simulink model "V_2_0_SystemsmModelling_ModifyAirCon"  (R2020a)
settings: Solver=ode23t  StartTime=0.0  StopTime=20000  MaxStep=2000.0  RelTol=1e-3
undefined symbols (not defined in the file or in its folder): building_height, building_length, building_width, Discrete, duct_area, fan_flow_rate_table, fan_setting_table, floor_conductivity, floor_heat_transfer_coeff_internal, floor_thickness, ground_temperature, initial_temperature, roof_conductivity, roof_density, roof_heat_transfer_coeff_external, roof_heat_transfer_coeff_internal, roof_specific_heat, roof_thickness, sigbuilder_block, Time, wall_conductivity, wall_density, wall_heat_transfer_coeff_external, wall_heat_transfer_coeff_internal, wall_specific_heat, wall_thickness
libraries: fl_lib x93, nesl_utility x16, simulink x1, ctrlSharedLib x1
(part 1 of 3)
settings Model: Creator=denni  LastModifiedBy=denni

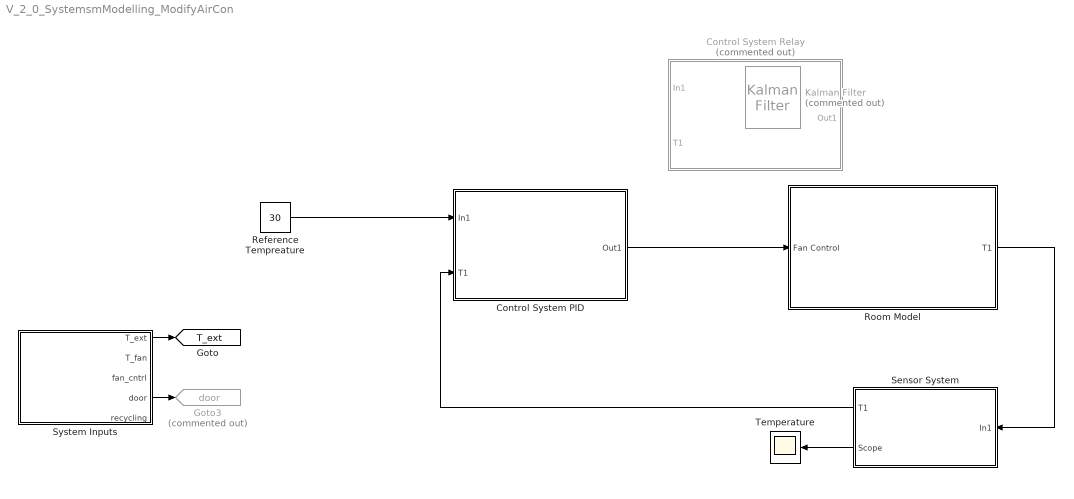
== system V_2_0_SystemsmModelling_ModifyAirCon ==
  Control System PID : Subsystem
  Control System Relay : Subsystem  Commented=on
  Goto3 : Goto  Commented=on  GotoTag=door  TagVisibility=global
  Kalman Filter : ctrlSharedLib/Kalman Filter  Commented=on  TimeDomain=Discrete-Time  UseCurrentEstimator=on  ModelSource=LTI State-Space Variable  ModelSourceVariable=ss(0.95,1,1,0,1)  A=0.95  B=1  C=1  D=0  NumberOfStates=1  NumberOfInputs=1  NumberOfOutputs=1  InitialEstimateSource=Dialog  X0=0  P0=10  UseK=off  UseGH=off  NumberOfProcessNoiseInputs=1  G=1  TimeInvariantG=on  H=0  TimeInvariantH=on  Q=0.05  TimeInvariantQ=on  R=1  TimeInvariantR=on  N=0  TimeInvariantN=on  AddInputPort=on  AddEnablePort=off  OutputEstimatedY=off  OutputP=off  Ts=-1
  "Reference Tempreature " : Constant  Value=30
  "Room Model " : Subsystem
  Sensor System : Subsystem
  System Inputs : Subsystem  Tag=STV Subsys  LoadFcn=sigbuilder_block('load');  StartFcn=sigbuilder_block('start');  StopFcn=sigbuilder_block('stop');  ClipboardFcn=sigbuilder_block('clipboard');  mask(Sigbuilder block){tuvar=[0:10]}
      mask help: Simulink:masks:SigbuilderBlock_MD
      mask init:
      | if ~strcmp(get_param(bdroot(gcbh),'SimulationStatus'),'stopped') tuvar = sigbuilder_block('maskInit'); end
      settings: CopyFcn=sigbuilder_block('copy');  DeleteFcn=sigbuilder_block('delete');  ModelCloseFcn=sigbuilder_block('modelClose');  PreSaveFcn=sigbuilder_block('preSave');  PauseFcn=sigbuilder_block('pause');  ContinueFcn=sigbuilder_block('continue');  NameChangeFcn=sigbuilder_block('namechange');  OpenFcn=sigbuilder_block('open',[334.8 172.8 550.8 361.2 ]);  CloseFcn=sigbuilder_block('close');
      mask Display: plot(0, 0, 100, 100,[2, 2, 32, 32, 2], [68, 8, 8, 68, 68],[32, 2], [38, 38], [32, 19, 2],[53, 60, 44], [32, 17, 17, 2],[16, 16, 31, 31]);txt = getActiveGroup(gcbh);text(2, 100, txt,'verticalAlignment', 'top');
  Temperature : Scope
  tag scope: T_ext=global
  wires:
  System Inputs/4(door) -> Goto3/1
  System Inputs/1(T_ext) -> [T_ext]
  "Room Model "/1(T1) -> Sensor System/1(In1)
  Sensor System/1(T1) -> Control System PID/2(T1)
  Sensor System/2(Scope) -> Temperature/1
  "Reference Tempreature "/1 -> Control System PID/1(In1)
  Control System PID/1(Out1) -> "Room Model "/1(Fan Control)

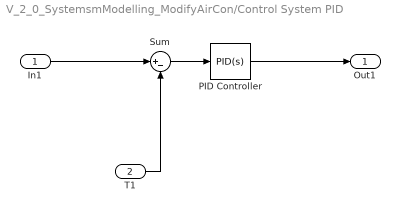
== system V_2_0_SystemsmModelling_ModifyAirCon/Control System PID ==
  In1 : Inport
  T1 : Inport  Port=2
  PID Controller : simulink/Continuous/PID Controller  Controller=PID  Form=Parallel  TimeDomain=Continuous-time  UseExternalTs=off  SampleTime=-1  IntegratorMethod=Forward Euler  FilterMethod=Forward Euler  ControllerParametersSource=internal  P=-0.718298192525533  I=-0.00178286353180639  D=22.2787509507692  UseFilter=on  N=0.00872543218655351  TunerSelectOption=Transfer Function Based (PID Tuner App)  InitialConditionSource=internal  InitialConditionForIntegrator=0  InitialConditionForFilter=0  DifferentiatorICPrevScaledInput=0  ExternalReset=none  TrackingMode=off  Kt=1  LimitOutput=off  UpperSaturationLimit=inf  LowerSaturationLimit=-inf  LinearizeAsGain=on  AntiWindupMode=none  Kb=1  POutMin=[]  POutMax=[]  IOutMin=[]  IOutMax=[]  DOutMin=[]  DOutMax=[]  NOutMin=[]  NOutMax=[]  SumOutMin=[]  SumOutMax=[]  SaturationOutMin=[]  SaturationOutMax=[]  PParamMin=[]  PParamMax=[]  IParamMin=[]  IParamMax=[]  DParamMin=[]  DParamMax=[]  NParamMin=[]  NParamMax=[]  KbParamMin=[]  KbParamMax=[]  KtParamMin=[]  KtParamMax=[]  KbOutMin=[]  KbOutMax=[]  KtOutMin=[]  KtOutMax=[]  IntegratorOutMin=[]  IntegratorOutMax=[]  FilterOutMin=[]  FilterOutMax=[]  SumI1OutMin=[]  SumI1OutMax=[]  SumI2OutMin=[]  SumI2OutMax=[]  SumI3OutMin=[]  SumI3OutMax=[]  SumI4OutMin=[]  SumI4OutMax=[]  SumDOutMin=[]  SumDOutMax=[]  DifferentiatorOutMin=[]  DifferentiatorOutMax=[]  FilterDiffOutCoefMin=[]  FilterDiffOutCoefMax=[]  ReciprocalOutMin=[]  ReciprocalOutMax=[]  SumDenOutMin=[]  SumDenOutMax=[]  SumNumOutMin=[]  SumNumOutMax=[]  DivideOutMin=[]  DivideOutMax=[]  UdiffTsProdOutMin=[]  UdiffTsProdOutMax=[]  NTsProdOutMin=[]  NTsProdOutMax=[]  UintegralTsProdOutMin=[]  UintegralTsProdOutMax=[]  UngainTsProdOutMin=[]  UngainTsProdOutMax=[]  IntegratorContinuousStateAttributes=''  IntegratorStateMustResolveToSignalObject=off  IntegratorRTWStateStorageClass=Auto  FilterContinuousStateAttributes=''  FilterStateMustResolveToSignalObject=off  FilterRTWStateStorageClass=Auto  ParallelPVariant=InternalParameters  IdealPVariant=Disabled  IVariant=InternalParameters  DVariant=InternalParameters  IntegratorVariant=Continuous  SatVariant=Disabled  AWVariant=Passthrough  PCopyVariant=Disabled  TRVariant=Disabled  FdbkBlocksVariant=Forward  IdealPFdbkVariant=Disabled  SatFdbkVariant=Disabled  DerivativeFilterVariant=ContFilter  NVariant=InternalParameters  NCopyVariant=Disabled  FilterICVariant=InternalICsFilter  IntegratorICVariant=InternalICs  ExternalResetVariant=Disabled  TRSumVariant=Passthrough  SumFdbkVariant=Disabled  SumVariant=Sum_PID  TsampFilterVariant=InternalTs  TsampNgainVariant=Passthrough  TsampIntegralVariant=Passthrough
  Sum : Sum  Inputs=|+-
  Out1 : Outport
  wires:
  In1/1 -> Sum/1
  T1/1 -> Sum/2
  Sum/1 -> PID Controller/1
  PID Controller/1 -> Out1/1

== system V_2_0_SystemsmModelling_ModifyAirCon/Control System Relay ==
  In1 : Inport
  T1 : Inport  Port=2
  Relay : Relay  OnSwitchValue=2  OffSwitchValue=-2
  Sum : Sum  Inputs=|-+
  Out1 : Outport
  wires:
  Sum/1 -> Relay/1
  Relay/1 -> Out1/1
  T1/1 -> Sum/2
  In1/1 -> Sum/1

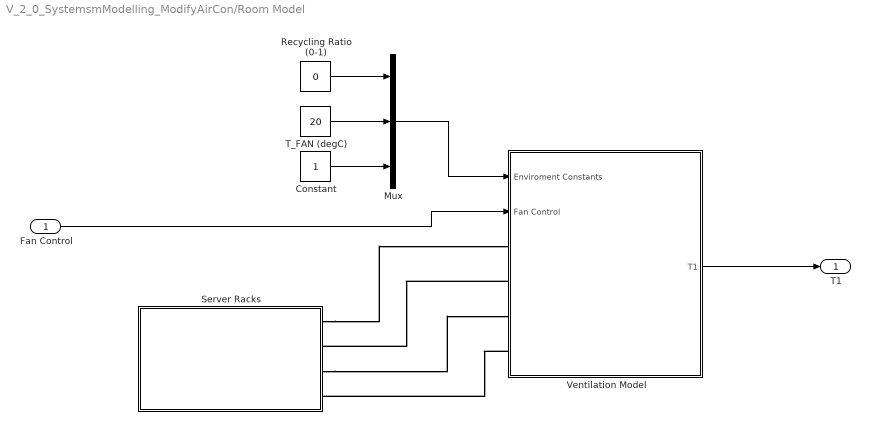
== system V_2_0_SystemsmModelling_ModifyAirCon/Room Model  ==
  Fan Control : Inport
  Constant : Constant
  Mux : Mux  Inputs=3
  Recycling Ratio (0-1) : Constant  Value=0
  Server Racks : Subsystem
  T_FAN (degC) : Constant  Value=20
  Ventilation Model : Subsystem
  T1 : Outport
  wires:
  Constant/1 -> Mux/3
  Recycling Ratio (0-1)/1 -> Mux/1
  T_FAN (degC)/1 -> Mux/2
  Mux/1 -> Ventilation Model/1(Enviroment Constants)
  Fan Control/1 -> Ventilation Model/2(Fan Control)
  Ventilation Model/1(T1) -> T1/1
  connections:
  Server Racks/LConn1 -- Ventilation Model/LConn1
  Ventilation Model/LConn2 -- Server Racks/LConn2
  Server Racks/LConn3 -- Ventilation Model/LConn3
  Ventilation Model/LConn4 -- Server Racks/LConn4

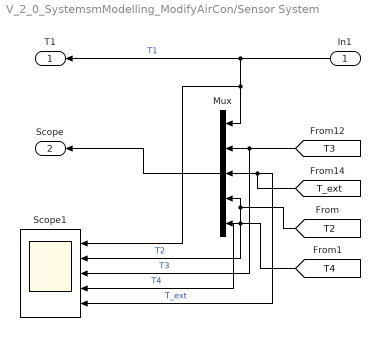
== system V_2_0_SystemsmModelling_ModifyAirCon/Sensor System ==
  In1 : Inport
  Mux : Mux  Inputs=5
  Scope1 : Scope  NumInputPorts=5
  T1 : Outport
  Scope : Outport  Port=2
  wires:
  [T3] -> Scope1/3, Mux/2  "T3"
  Mux/1 -> Scope/1
  [T_ext] -> Mux/3, Scope1/5  "T_ext"
  In1/1 -> Mux/1, Scope1/1, T1/1  "T1"
  [T4] -> Scope1/4, Mux/5  "T4"
  [T2] -> Mux/4, Scope1/2  "T2"

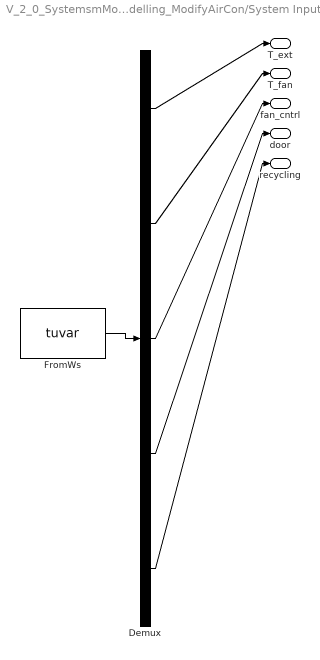
== system V_2_0_SystemsmModelling_ModifyAirCon/System Inputs ==
  Demux : Demux  Tag=STV Demux  Outputs=5
      settings: DisplayOption=none
  FromWs : FromWorkspace  Tag=STV FromWs  VariableName=tuvar
      SigBuilderData=|
      | common.afterFinalStr = 'Extrapolate'
      | common.sampleTime = 0
      | dataSet(1).timeRange = [0 100000]
      | dataSet(1).name = 'Fan Control'
      | dataSet(2).timeRange = [0 100000]
      | dataSet(2).name = 'Fan Temperature'
      | dataSet(3).timeRange = [0 100000]
      | dataSet(3).name = 'Disturbances'
      | sbobj.Groups(1).Name = 'Fan Control'
      | sbobj.Groups(1).Signals(1).Name = 'T_ext'
      | sbobj.Groups(1).Signals(1).XData = [0 100000]
      | sbobj.Groups(1).Signals(1).YData = [35 35]
      | sbobj.Groups(1).Signals(2).Name = 'T_fan'
      | sbobj.Groups(1).Signals(2).XData = [0 100000]
      | sbobj.Groups(1).Signals(2).YData = [20.05 20.05]
      | sbobj.Groups(1).Signals(3).Name = 'fan_cntrl'
      | sbobj.Groups(1).Signals(3).XData = [0 20000 20000 40000 60000 80000 100000]
      | sbobj.Groups(1).Signals(3).YData = [1.1 1.1 1.04 1.04 1.04 1.04 1.04]
      | sbobj.Groups(1).Signals(4).Name = 'door'
      | sbobj.Groups(1).Signals(4).XData = [0 100000]
      | sbobj.Groups(1).Signals(4).YData = [0 0]
      | sbobj.Groups(1).Signals(5).Name = 'recycling'
      | sbobj.Groups(1).Signals(5).XData = [0 100000]
      | sbobj.Groups(1).Signals(5).YData = [0 0]
      | sbobj.Groups(1).TimeRange = [0 100000]
      | sbobj.Groups(2).Name = 'Fan Temperature'
      | sbobj.Groups(2).Signals(1).Name = 'T_ext'
      | sbobj.Groups(2).Signals(1).XData = [0 100000]
      | sbobj.Groups(2).Signals(1).YData = [35 35]
      | sbobj.Groups(2).Signals(2).Name = 'T_fan'
      | sbobj.Groups(2).Signals(2).XData = [0 20000 20000 40000 40000 60000 60000 80000 80000 100000]
      | sbobj.Groups(2).Signals(2).YData = [20 20 15 15 20 20 35 35 20 20]
      | sbobj.Groups(2).Signals(3).Name = 'fan_cntrl'
      | sbobj.Groups(2).Signals(3).XData = [0 100000]
      | sbobj.Groups(2).Signals(3).YData = [1 1]
      | sbobj.Groups(2).Signals(4).Name = 'door'
      | sbobj.Groups(2).Signals(4).XData = [0 100000]
      | sbobj.Groups(2).Signals(4).YData = [0 0]
      | sbobj.Groups(2).Signals(5).Name = 'recycling'
      | sbobj.Groups(2).Signals(5).XData = [0 100000]
      | sbobj.Groups(2).Signals(5).YData = [0 0]
      | sbobj.Groups(2).TimeRange = [0 100000]
      | sbobj.Groups(3).Name = 'Disturbances'
      | sbobj.Groups(3).Signals(1).Name = 'T_ext'
      | sbobj.Groups(3).Signals(1).XData = [0 100000]
      | sbobj.Groups(3).Signals(1).YData = [35 35]
      | sbobj.Groups(3).Signals(2).Name = 'T_fan'
      | sbobj.Groups(3).Signals(2).XData = [0 100000]
      | sbobj.Groups(3).Signals(2).YData = [20 20]
      | sbobj.Groups(3).Signals(3).Name = 'fan_cntrl'
      | sbobj.Groups(3).Signals(3).XData = [0 100000]
      | sbobj.Groups(3).Signals(3).YData = [1 1]
      | sbobj.Groups(3).Signals(4).Name = 'door'
      | sbobj.Groups(3).Signals(4).XData = [0 20000 30000 40000 100000]
      | sbobj.Groups(3).Signals(4).YData = [0 0 1 0 0]
      | sbobj.Groups(3).Signals(5).Name = 'recycling'
      | sbobj.Groups(3).Signals(5).XData = [0 60000 60000 80000 80000 100000]
      | sbobj.Groups(3).Signals(5).YData = [0 0 0.5 0.5 0 0]
      | sbobj.Groups(3).TimeRange = [0 100000]
  T_ext : Outport  Tag=STV Outport  VectorParamsAs1DForOutWhenUnconnected=off
  T_fan : Outport  Tag=STV Outport  Port=2  VectorParamsAs1DForOutWhenUnconnected=off
  fan_cntrl : Outport  Tag=STV Outport  Port=3  VectorParamsAs1DForOutWhenUnconnected=off
  door : Outport  Tag=STV Outport  Port=4  VectorParamsAs1DForOutWhenUnconnected=off
  recycling : Outport  Tag=STV Outport  Port=5  VectorParamsAs1DForOutWhenUnconnected=off
  wires:
  FromWs/1 -> Demux/1
  Demux/1 -> T_ext/1
  Demux/2 -> T_fan/1
  Demux/3 -> fan_cntrl/1
  Demux/4 -> door/1
  Demux/5 -> recycling/1

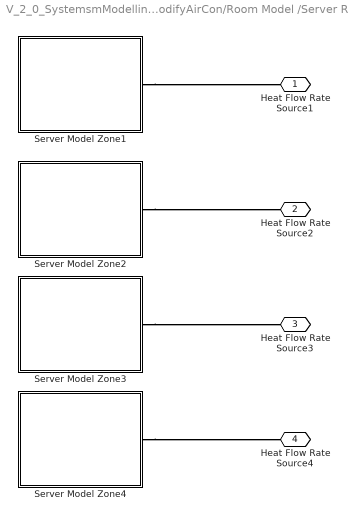
== system V_2_0_SystemsmModelling_ModifyAirCon/Room Model /Server Racks ==
  Server Model Zone1 : Subsystem
  Server Model Zone2 : Subsystem
  Server Model Zone3 : Subsystem
  Server Model Zone4 : Subsystem
  Heat Flow Rate Source1 : PMIOPort  Side=Left
  Heat Flow Rate Source2 : PMIOPort  Port=2  Side=Left
  Heat Flow Rate Source3 : PMIOPort  Port=3  Side=Left
  Heat Flow Rate Source4 : PMIOPort  Port=4  Side=Left
  connections:
  Server Model Zone2/LConn1 -- Heat Flow Rate Source2/RConn1
  Server Model Zone1/LConn1 -- Heat Flow Rate Source1/RConn1
  Server Model Zone4/LConn1 -- Heat Flow Rate Source4/RConn1
  Server Model Zone3/LConn1 -- Heat Flow Rate Source3/RConn1
